simulink model "Controller_cirrus"  (R2024b)
settings: Solver=VariableStepAuto  StartTime=0.0  StopTime=10.0  RelTol=1e-3
undefined symbols (not defined in the file): states_init
libraries: slpidlib x4, simulink_extras x2
settings Model: Creator=nicom  LastModifiedBy=nicom

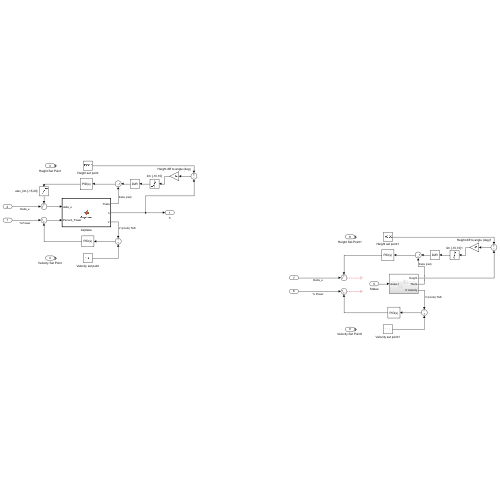
[thumbnail: Simulink's stored preview of the top-level diagram]
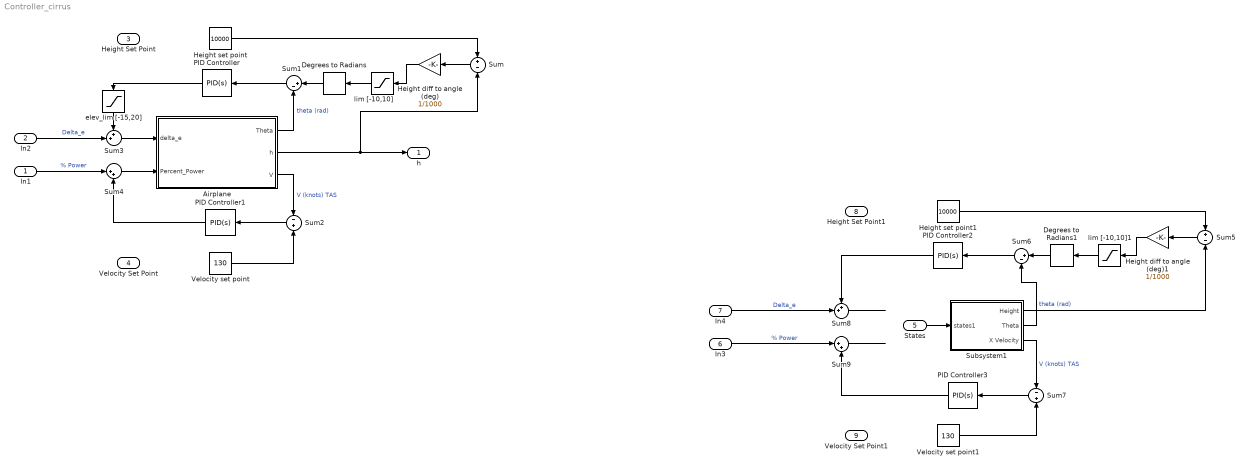
== system Controller_cirrus ==
  In1 : Inport
  In2 : Inport  Port=2
  Height Set Point : Inport  Port=3
  Velocity Set Point : Inport  Port=4
  States : Inport  Port=5
  In3 : Inport  Port=6
  In4 : Inport  Port=7
  Height Set Point1 : Inport  Port=8
  Velocity Set Point1 : Inport  Port=9
  Airplane : MATLAB Function  TreatAsAtomicUnit=on
  Degrees to Radians : simulink_extras/Transformations/Degrees to Radians
  Degrees to Radians1 : simulink_extras/Transformations/Degrees to Radians
  Height diff to angle (deg) : Gain  Gain=1/1000
  Height diff to angle (deg)1 : Gain  Gain=1/1000
  Height set point : Constant  Value=10000
  Height set point1 : Constant  Value=10000
  PID Controller{,1..3} (4 alike) : slpidlib/PID Controller  Controller=PID  Form=Parallel  TimeDomain=Continuous-time  UseExternalTs=off  SampleTime=-1  IntegratorMethod=Forward Euler  FilterMethod=Forward Euler  ControllerParametersSource=internal  P=1  I=1  UseKiTs=off  D=0  UseExternalDerivativeSource=off  N=100  UseFilter=on  TunerSelectOption=Transfer Function Based (PID Tuner App)  InitialConditionSource=internal  InitialConditionForIntegrator=0  InitialConditionForFilter=0  DifferentiatorICPrevScaledInput=0  ExternalReset=none  TrackingMode=off  Kt=1  LimitOutput=off  SatLimitsSource=internal  UpperSaturationLimit=inf  LowerSaturationLimit=-inf  LinearizeAsGain=on  AntiWindupMode=none  Kb=1  LimitIntegrator=off  UpperIntegratorSaturationLimit=inf  LowerIntegratorSaturationLimit=-inf  POutMin=[]  POutMax=[]  IOutMin=[]  IOutMax=[]  DOutMin=[]  DOutMax=[]  NOutMin=[]  NOutMax=[]  SumOutMin=[]  SumOutMax=[]  SaturationOutMin=[]  SaturationOutMax=[]  PParamMin=[]  PParamMax=[]  IParamMin=[]  IParamMax=[]  DParamMin=[]  DParamMax=[]  NParamMin=[]  NParamMax=[]  KbParamMin=[]  KbParamMax=[]  KtParamMin=[]  KtParamMax=[]  KbOutMin=[]  KbOutMax=[]  KtOutMin=[]  KtOutMax=[]  IntegratorOutMin=[]  IntegratorOutMax=[]  FilterOutMin=[]  FilterOutMax=[]  SumI1OutMin=[]  SumI1OutMax=[]  SumI2OutMin=[]  SumI2OutMax=[]  SumI3OutMin=[]  SumI3OutMax=[]  SumI4OutMin=[]  SumI4OutMax=[]  SumDOutMin=[]  SumDOutMax=[]  DifferentiatorOutMin=[]  DifferentiatorOutMax=[]  FilterDiffOutCoefMin=[]  FilterDiffOutCoefMax=[]  ReciprocalOutMin=[]  ReciprocalOutMax=[]  SumDenOutMin=[]  SumDenOutMax=[]  SumNumOutMin=[]  SumNumOutMax=[]  DivideOutMin=[]  DivideOutMax=[]  UdiffTsProdOutMin=[]  UdiffTsProdOutMax=[]  NTsProdOutMin=[]  NTsProdOutMax=[]  UintegralTsProdOutMin=[]  UintegralTsProdOutMax=[]  UngainTsProdOutMin=[]  UngainTsProdOutMax=[]  ClampingZeroOutDataTypeStr=Inherit: Inherit via back propagation  ClampingZeroOutMin=[]  ClampingZeroOutMax=[]  FilterDenConstantOutDataTypeStr=Inherit: Inherit via back propagation  FilterDenConstantOutMin=[]  FilterDenConstantOutMax=[]  PCopyOutDataTypeStr=Inherit: Inherit via back propagation  PCopyOutMin=[]  PCopyOutMax=[]  NCopyOutDataTypeStr=Inherit: Inherit via back propagation  NCopyOutMin=[]  NCopyOutMax=[]  IntegratorContinuousStateAttributes=''  IntegratorStateMustResolveToSignalObject=off  IntegratorRTWStateStorageClass=Auto  FilterContinuousStateAttributes=''  FilterStateMustResolveToSignalObject=off  FilterRTWStateStorageClass=Auto  ParallelPVariant=InternalParameters  IdealPVariant=Disabled  IVariant=InternalParameters  DVariant=InternalParameters  IntegratorVariant=Continuous  SatVariant=Disabled  AWVariant=Passthrough  PCopyVariant=Disabled  TRVariant=Disabled  FdbkBlocksVariant=Forward  IdealPFdbkVariant=Disabled  SatFdbkVariant=Disabled  DerivativeFilterVariant=ContFilter  NVariant=InternalParameters  NCopyVariant=Disabled  FilterICVariant=InternalICsFilter  IntegratorICVariant=InternalICs  ExternalResetVariant=Disabled  TRSumVariant=Passthrough  SumFdbkVariant=Disabled  SumVariant=Sum_PID  TsampFilterVariant=InternalTs  TsampNgainVariant=Passthrough  TsampIntegralVariant=Disabled_SignalSpec  ExternalSaturationOutDataTypeStr=Inherit: Same as second input  DerivativeSourceVariant=ErrorSignal  PreIntVariant=InternalPreInt
  Subsystem1 : Subsystem
  Sum : Sum  Inputs=+|-
  Sum1 : Sum  Inputs=|+-
  Sum2 : Sum  Inputs=-|+
  Sum3 : Sum  Inputs=++|
  Sum4 : Sum  Inputs=|++
  Sum5 : Sum  Inputs=+|-
  Sum6 : Sum  Inputs=|+-
  Sum7 : Sum  Inputs=-|+
  Sum8 : Sum  Inputs=++|
  Sum9 : Sum  Inputs=|++
  Velocity set point : Constant  Value=130
  Velocity set point1 : Constant  Value=130
  elev_lim [-15,20] : Saturate  UpperLimit=25  LowerLimit=-15
  lim [-10,10] : Saturate  UpperLimit=10  LowerLimit=-10
  lim [-10,10]1 : Saturate  UpperLimit=10  LowerLimit=-10
  h : Outport
  wires:
  Height set point/1 -> Sum/1
  Airplane/1(Theta) -> Sum1/2  "theta (rad)"
  Airplane/2(h) -> Sum/2, h/1
  Sum1/1 -> PID Controller/1
  Airplane/3(V) -> Sum2/1  "V (knots) TAS"
  Sum2/1 -> PID Controller1/1
  Velocity set point/1 -> Sum2/2
  PID Controller/1 -> elev_lim [-15,20]/1
  PID Controller1/1 -> Sum4/2
  Sum3/1 -> Airplane/1(delta_e)
  Sum4/1 -> Airplane/2(Percent_Power)
  In2/1 -> Sum3/2  "Delta_e"
  In1/1 -> Sum4/1  "% Power"
  Sum/1 -> Height diff to angle (deg)/1
  Height diff to angle (deg)/1 -> lim [-10,10]/1
  Degrees to Radians/1 -> Sum1/1
  lim [-10,10]/1 -> Degrees to Radians/1
  elev_lim [-15,20]/1 -> Sum3/1
  Height diff to angle (deg)1/1 -> lim [-10,10]1/1
  lim [-10,10]1/1 -> Degrees to Radians1/1
  In4/1 -> Sum8/2  "Delta_e"
  Height set point1/1 -> Sum5/1
  Subsystem1/1(Height) -> Sum5/2
  Subsystem1/3(X Velocity) -> Sum7/1  "V (knots) TAS"
  Sum7/1 -> PID Controller3/1
  Sum6/1 -> PID Controller2/1
  Subsystem1/2(Theta) -> Sum6/2  "theta (rad)"
  Sum5/1 -> Height diff to angle (deg)1/1
  PID Controller3/1 -> Sum9/2
  States/1 -> Subsystem1/1(states1)
  Velocity set point1/1 -> Sum7/2
  PID Controller2/1 -> Sum8/1
  Sum8/1 -> ?
  Degrees to Radians1/1 -> Sum6/1
  In3/1 -> Sum9/1  "% Power"
  Sum9/1 -> ?

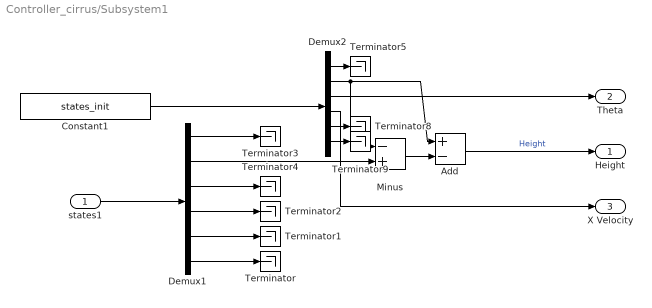
== system Controller_cirrus/Subsystem1 ==
  states1 : Inport
  Add : Sum  Inputs=+-
  Constant1 : Constant  Value=states_init
  Demux1 : Demux  Outputs=6
  Demux2 : Demux  Outputs=6
  Minus : Sum  Inputs=-+
  Terminator{,1..5,8..9} (8 alike) : Terminator
  Height : Outport
  Theta : Outport  Port=2
  X Velocity : Outport  Port=3
  wires:
  Constant1/1 -> Demux2/1
  Demux1/3 -> Terminator4/1
  Demux1/4 -> Terminator2/1
  Demux1/1 -> Terminator3/1
  Demux2/6 -> Terminator9/1
  Demux1/2 -> Minus/2
  states1/1 -> Demux1/1
  Demux1/6 -> Terminator/1
  Demux1/5 -> Terminator1/1
  Demux2/2 -> Add/1, Minus/1
  Minus/1 -> Add/2
  Add/1 -> Height/1  "Height"
  Demux2/3 -> Theta/1
  Demux2/1 -> Terminator5/1
  Demux2/5 -> Terminator8/1
  Demux2/4 -> X Velocity/1

== matlab function Controller_cirrus/Airplane ==
  data: delta_e input; Theta output; h output; V output; Percent_Power input
function [Theta, h, V] = Airplane(delta_e, Percent_Power)
